simulink model "encoder_sim"  (R2015a)
settings: Solver=FixedStepDiscrete  StartTime=0.0  StopTime=60  RelTol=1e-3
libraries: arduino_io_lib x4
settings Model: Creator=gcampa  LastModifiedBy=Osman
settings DataIOCC: SignalLoggingSaveFormat=ModelDataLogs
settings OptimizationCC: ExpressionDepthLimit=2147483647
settings DebuggingCC: UnderspecifiedInitializationDetection=Classic  MergeDetectMultiDrivingBlocksExec=none  SolverPrmCheckMsg=warning  FcnCallInpInsideContextMsg=UseLocalSettings  StateNameClashWarn=warning
settings GRTTargetCC: CombineOutputUpdateFcns=off  GRTInterface=on

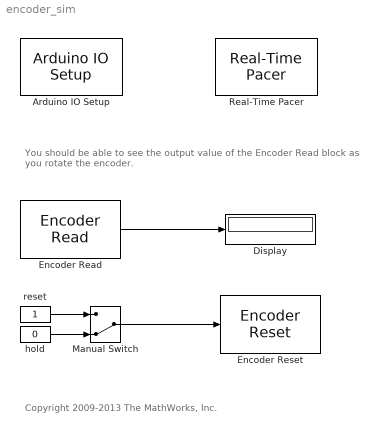
== system encoder_sim ==
  note: You should be able to see the output value of the Encoder Read
      | block as you rotate the encoder.
  note: Copyright 2009-2013 The MathWorks, Inc.
  Arduino IO Setup : arduino_io_lib/Arduino IO Setup  Priority=3  arduinoVar=Temporary arduino variable: Arduino2  workspaceVarName=b  comPort=COM17
  Display : Display
  Encoder Read : arduino_io_lib/Encoder Read  arduinoVar=Temporary arduino variable: Arduino2  encNum=1  pinA=3  pinB=2  DbDl=17  T=0.2
  Encoder Reset : arduino_io_lib/Encoder Reset  arduinoVar=Temporary arduino variable: Arduino2  encNum=1  T=0.2
  Manual Switch : ManualSwitch  CurrentSetting=0
  Real-Time Pacer : arduino_io_lib/Real-Time Pacer  simTimePerRealTime=1
  hold : Constant  Value=0
  reset : Constant
  wires:
  Encoder Read/1 -> Display/1
  reset/1 -> Manual Switch/1
  hold/1 -> Manual Switch/2
  Manual Switch/1 -> Encoder Reset/1
